simulink model "practise3"  (R2017b)
settings: Solver=VariableStepAuto  StartTime=0.0  StopTime=10.0  RelTol=1e-3
values from neighbouring files (symbols this model uses):
  Ce = max(u)/B    [pract3.m]
  J = tau2*Ce^2/R    [pract3.m]
  R = (max(u)+B*Ce)/A    [pract3.m]
libraries: fl_lib x11, nesl_utility x8
settings Model: Creator=Aleksandr  LastModifiedBy=Aleksandr

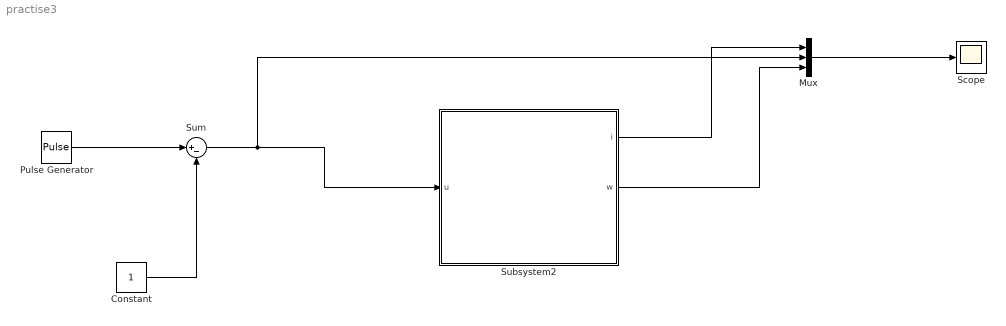
== system practise3 ==
  Constant : Constant
  Mux : Mux  Inputs=3
  Pulse Generator : DiscretePulseGenerator  PulseType=Time based  Amplitude=2  Period=5  PulseWidth=50
  Scope : Scope
  Subsystem2 : Subsystem
  Sum : Sum  Inputs=|+-
  wires:
  Pulse Generator/1 -> Sum/1
  Constant/1 -> Sum/2
  Sum/1 -> Mux/2, Subsystem2/1(u)
  Mux/1 -> Scope/1
  Subsystem2/1(i) -> Mux/1
  Subsystem2/2(w) -> Mux/3

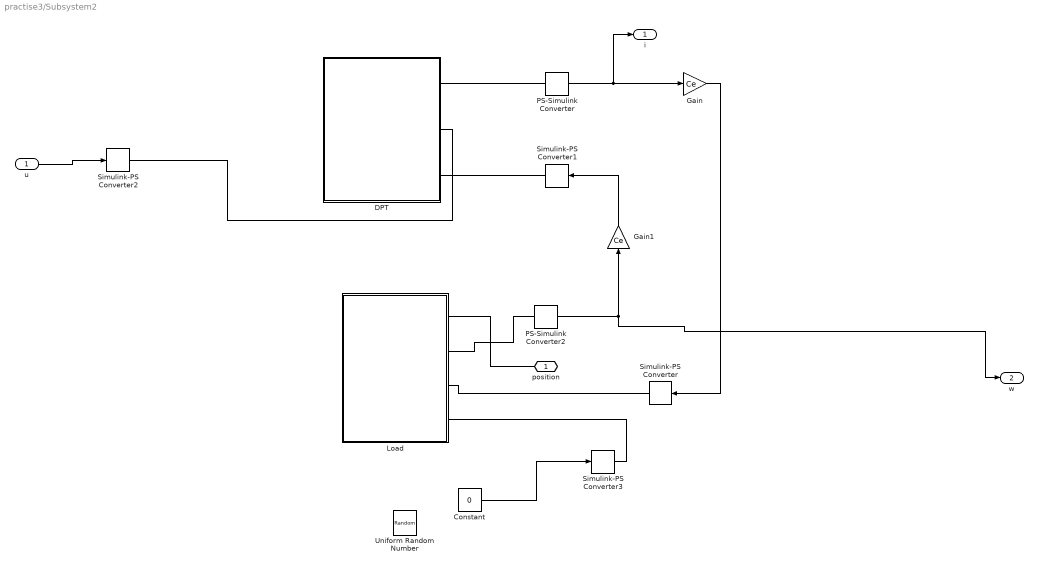
== system practise3/Subsystem2 ==
  u : Inport
  Constant : Constant  Value=0
  DPT : Subsystem
  Gain : Gain  Gain=Ce
  Gain1 : Gain  Gain=Ce
  Load : Subsystem
  PS-Simulink Converter : nesl_utility/PS-Simulink Converter  PhysicalDomain=network_engine_domain  SubClassName=ps_output  LeftPortType=input  RightPortType=output  PseudoPeriodic=off  Frequencies=[]  Unit=1  AffineConversion=off
  PS-Simulink Converter2 : nesl_utility/PS-Simulink Converter  PhysicalDomain=network_engine_domain  SubClassName=ps_output  LeftPortType=input  RightPortType=output  PseudoPeriodic=off  Frequencies=[]  Unit=1  AffineConversion=off
  Simulink-PS Converter : nesl_utility/Simulink-PS Converter  PhysicalDomain=network_engine_domain  SubClassName=ps_input  LeftPortType=input  RightPortType=output  PseudoPeriodic=off  Frequencies=[]  NoiseDistribution=none  NoiseParameters=[]  Unit=1  AffineConversion=off  FilteringAndDerivatives=provide  SimscapeFilterOrder=2  InputFilterTimeConstant=0.001  UdotUserProvided=0
  Simulink-PS Converter1 : nesl_utility/Simulink-PS Converter  PhysicalDomain=network_engine_domain  SubClassName=ps_input  LeftPortType=input  RightPortType=output  PseudoPeriodic=off  Frequencies=[]  NoiseDistribution=none  NoiseParameters=[]  Unit=1  AffineConversion=off  FilteringAndDerivatives=provide  SimscapeFilterOrder=2  InputFilterTimeConstant=0.001  UdotUserProvided=0
  Simulink-PS Converter2 : nesl_utility/Simulink-PS Converter  PhysicalDomain=network_engine_domain  SubClassName=ps_input  LeftPortType=input  RightPortType=output  PseudoPeriodic=off  Frequencies=[]  NoiseDistribution=none  NoiseParameters=[]  Unit=1  AffineConversion=off  FilteringAndDerivatives=provide  SimscapeFilterOrder=2  InputFilterTimeConstant=0.001  UdotUserProvided=0
  Simulink-PS Converter3 : nesl_utility/Simulink-PS Converter  PhysicalDomain=network_engine_domain  SubClassName=ps_input  LeftPortType=input  RightPortType=output  PseudoPeriodic=off  Frequencies=[]  NoiseDistribution=none  NoiseParameters=[]  Unit=1  AffineConversion=off  FilteringAndDerivatives=provide  SimscapeFilterOrder=1  InputFilterTimeConstant=0.001  UdotUserProvided=0
  Uniform Random Number : UniformRandomNumber  Minimum=-0.1  Maximum=0.1  SampleTime=0.1
  position : PMIOPort  Port=1  Side=Right
  i : Outport
  w : Outport  Port=2
  wires:
  PS-Simulink Converter/1 -> Gain/1, i/1
  Gain/1 -> Simulink-PS Converter/1
  PS-Simulink Converter2/1 -> w/1, Gain1/1
  Gain1/1 -> Simulink-PS Converter1/1
  u/1 -> Simulink-PS Converter2/1
  Constant/1 -> Simulink-PS Converter3/1
  connections:
  PS-Simulink Converter/LConn1 -- DPT/RConn1
  Load/RConn3 -- Simulink-PS Converter/RConn1
  Simulink-PS Converter1/RConn1 -- DPT/RConn3
  position/RConn1 -- Load/RConn1
  PS-Simulink Converter2/LConn1 -- Load/RConn2
  Simulink-PS Converter3/RConn1 -- Load/RConn4
  Simulink-PS Converter2/RConn1 -- DPT/RConn2

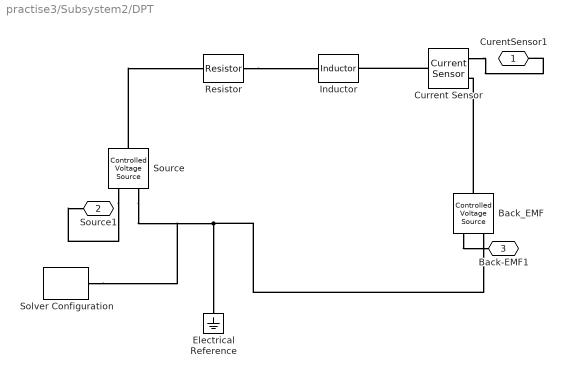
== system practise3/Subsystem2/DPT ==
  Back_EMF : fl_lib/Electrical/Electrical Sources/Controlled Voltage Source
  Current Sensor : fl_lib/Electrical/Electrical Sensors/Current Sensor
  Electrical Reference : fl_lib/Electrical/Electrical Elements/Electrical Reference
  Inductor : fl_lib/Electrical/Electrical Elements/Inductor  l=L H  r=0 Ohm  g=1e-9 1/Ohm  i_specify=off  i_priority=None  i=0 A  i_nominal_specify=off  i_nominal_unit=A  i_nominal_value=1  v_specify=off  v_priority=None  v=0 V  v_nominal_specify=off  v_nominal_unit=V  v_nominal_value=1  i_L_specify=off  i_L_priority=High  i_L=0 A  i_L_nominal_specify=off  i_L_nominal_unit=A  i_L_nominal_value=1
  Resistor : fl_lib/Electrical/Electrical Elements/Resistor  R=R Ohm  i_specify=off  i_priority=None  i=0 A  i_nominal_specify=off  i_nominal_unit=A  i_nominal_value=1  v_specify=off  v_priority=None  v=0 V  v_nominal_specify=off  v_nominal_unit=V  v_nominal_value=1
  Solver Configuration : nesl_utility/Solver Configuration  PhysicalDomain=network_engine_domain  SubClassName=solver  LeftPortType=input  RightPortType=generic  Accelerate=off  Tones=[]  Harmonics=[]  SimulateNoise=off  Profile=off  UseLocalSampling=off  EnableSwitchedLinearOptims=on  FrequencyDomain=off  UseCCode=off  RelTol=0.001  AbsTol=1e-06  MinStep=1e-09  ToWorkspace=off  RevertToSquareIcSolve=off  NumHomotopyIterations=100  PhasorMode=off  PhasorModeNumHarmonics=1  DoDC=off  ResidualTolerance=1e-09  UseLocalSolver=off  LocalSolverChoice=NE_BACKWARD_EULER_ADVANCER  LocalSolverSampleTime=0.001  DoFixedCost=off  MaxNonlinIter=3  MaxModeIter=2  LinearAlgebra=Sparse  DelaysMemoryBudget=1024  AutomaticFiltering=on  FilteringTimeConstant=0.001
  Source : fl_lib/Electrical/Electrical Sources/Controlled Voltage Source
  CurentSensor1 : PMIOPort  Port=1  Side=Right
  Source1 : PMIOPort  Port=2  Side=Right
  Back-EMF1 : PMIOPort  Port=3  Side=Right
  connections:
  Resistor/RConn1 -- Inductor/LConn1
  Back_EMF/RConn2 -- Solver Configuration/RConn1 -- Source/RConn2 -- Electrical Reference/LConn1
  Source/LConn1 -- Resistor/LConn1
  Current Sensor/LConn1 -- Inductor/RConn1
  Back_EMF/LConn1 -- Current Sensor/RConn2
  Back_EMF/RConn1 -- Back-EMF1/RConn1
  Current Sensor/RConn1 -- CurentSensor1/RConn1
  Source/RConn1 -- Source1/RConn1

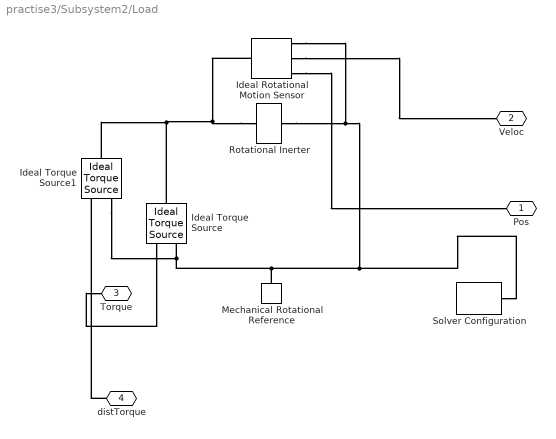
== system practise3/Subsystem2/Load ==
  Ideal Rotational Motion Sensor : fl_lib/Mechanical/Mechanical Sensors/Ideal Rotational Motion Sensor  offset=0 rad
  Ideal Torque Source : fl_lib/Mechanical/Mechanical Sources/Ideal Torque Source
  Ideal Torque Source1 : fl_lib/Mechanical/Mechanical Sources/Ideal Torque Source
  Mechanical Rotational Reference : fl_lib/Mechanical/Rotational Elements/Mechanical Rotational Reference
  Rotational Inerter : fl_lib/Mechanical/Rotational Elements/Rotational Inerter  B=J kg*m^2  w_specify=off  w_priority=High  w=0 rad/s  w_nominal_specify=off  w_nominal_unit=rad/s  w_nominal_value=1  t_specify=off  t_priority=None  t=0 N*m  t_nominal_specify=off  t_nominal_unit=N*m  t_nominal_value=1
      settings: SourceProductName=Simscape  SourceProductBaseCode=SS
  Solver Configuration : nesl_utility/Solver Configuration  PhysicalDomain=network_engine_domain  SubClassName=solver  LeftPortType=input  RightPortType=generic  Accelerate=off  Tones=[]  Harmonics=[]  SimulateNoise=off  Profile=off  UseLocalSampling=off  EnableSwitchedLinearOptims=on  FrequencyDomain=off  UseCCode=off  RelTol=0.001  AbsTol=1e-06  MinStep=1e-09  ToWorkspace=off  RevertToSquareIcSolve=off  NumHomotopyIterations=100  PhasorMode=off  PhasorModeNumHarmonics=1  DoDC=off  ResidualTolerance=1e-09  UseLocalSolver=off  LocalSolverChoice=NE_BACKWARD_EULER_ADVANCER  LocalSolverSampleTime=0.001  DoFixedCost=off  MaxNonlinIter=3  MaxModeIter=2  LinearAlgebra=Sparse  DelaysMemoryBudget=1024  AutomaticFiltering=on  FilteringTimeConstant=0.001
  Pos : PMIOPort  Port=1  Side=Right
  Veloc : PMIOPort  Port=2  Side=Right
  Torque : PMIOPort  Port=3  Side=Right
  distTorque : PMIOPort  Port=4  Side=Right
  connections:
  Ideal Rotational Motion Sensor/RConn2 -- Veloc/RConn1
  Ideal Rotational Motion Sensor/RConn3 -- Pos/RConn1
  Ideal Torque Source/RConn1 -- Torque/RConn1
  Ideal Torque Source/RConn2 -- Mechanical Rotational Reference/LConn1 -- Solver Configuration/RConn1 -- Rotational Inerter/RConn1 -- Ideal Rotational Motion Sensor/RConn1 -- Ideal Torque Source1/RConn2
  Rotational Inerter/LConn1 -- Ideal Rotational Motion Sensor/LConn1 -- Ideal Torque Source/LConn1 -- Ideal Torque Source1/LConn1
  distTorque/RConn1 -- Ideal Torque Source1/RConn1
